simulink model "hw2_skml"  (R2024a)
settings: Solver=VariableStepAuto  StartTime=0.0  StopTime=10.0  RelTol=1e-3
settings Model: Creator=s14  LastModifiedBy=s14

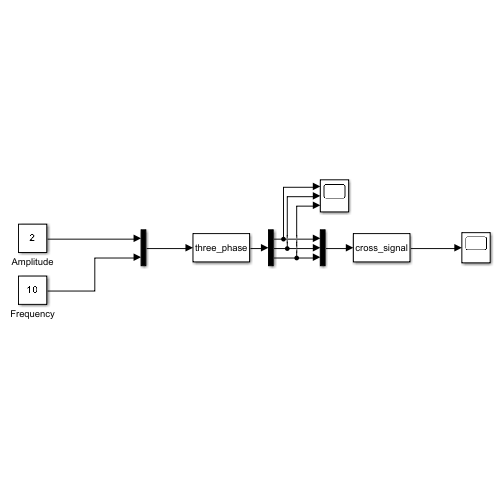
[thumbnail: Simulink's stored preview of the top-level diagram]
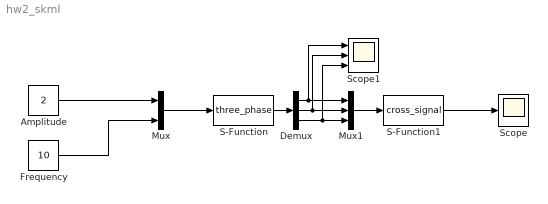
== system hw2_skml ==
  Amplitude : Constant  Value=2
  Demux : Demux  Outputs=3
  Frequency : Constant  Value=10
  Mux : Mux  Inputs=2
  Mux1 : Mux  Inputs=3
  S-Function : S-Function  FunctionName=three_phase  SFunctionDeploymentMode=off  EnableBusSupport=off
  S-Function1 : S-Function  FunctionName=cross_signal  SFunctionDeploymentMode=off  EnableBusSupport=off
  Scope : Scope
  Scope1 : Scope  NumInputPorts=3
  wires:
  Mux/1 -> S-Function/1
  Amplitude/1 -> Mux/1
  Frequency/1 -> Mux/2
  S-Function/1 -> Demux/1
  Mux1/1 -> S-Function1/1
  Demux/1 -> Scope1/1, Mux1/1
  Demux/2 -> Scope1/2, Mux1/2
  Demux/3 -> Scope1/3, Mux1/3
  S-Function1/1 -> Scope/1
